simulink model "UDPVarFrameTest"  (R2013b)
settings: Solver=ode1  StartTime=0.0  StopTime=300  FixedStep=simPars.SampleTime  RelTol=1e-3
undefined symbols (not defined in the file or in its folder): simPars
libraries: instrumentlib x2, etargetslib x1
settings Model: Creator=Paul Freeman  LastModifiedBy=descobar
settings DataIOCC: LimitDataPoints=off  SignalLoggingSaveFormat=ModelDataLogs  SaveOutput=off  SignalLogging=off
settings OptimizationCC: ExpressionDepthLimit=2147483647
settings DebuggingCC: FcnCallInpInsideContextMsg=UseLocalSettings  StateNameClashWarn=warning
settings HardwareCC: ProdLargestAtomicInteger=Long  ProdLargestAtomicFloat=Double  ProdIntDivRoundTo=Zero  ProdEndianess=BigEndian  ProdHWDeviceType=Freescale->32-bit PowerPC
settings SFSimCC: SimParseCustomCode=off
settings GRTTargetCC: CombineOutputUpdateFcns=off  GRTInterface=on

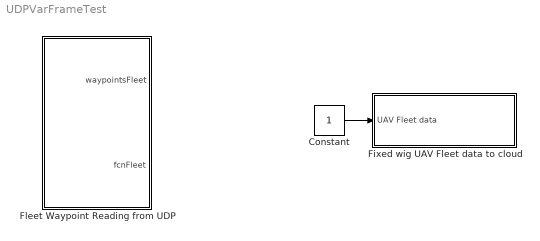
== system UDPVarFrameTest ==
  Constant : Constant
  Fixed wig UAV Fleet data to cloud : Subsystem
  Fleet Waypoint Reading from UDP : Subsystem
  wires:
  Constant/1 -> Fixed wig UAV Fleet data to cloud/1(UAV Fleet data)

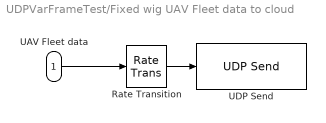
== system UDPVarFrameTest/Fixed wig UAV Fleet data to cloud ==
  UAV Fleet data : Inport
  Rate Transition : RateTransition  OutPortSampleTime=simPars.SampleTime*5
  UDP Send : instrumentlib/UDP Send  Host=localhost  Port=5556  LocalPort=5556  EnableBlockingMode=on  ByteOrder=BigEndian
  wires:
  Rate Transition/1 -> UDP Send/1
  UAV Fleet data/1 -> Rate Transition/1

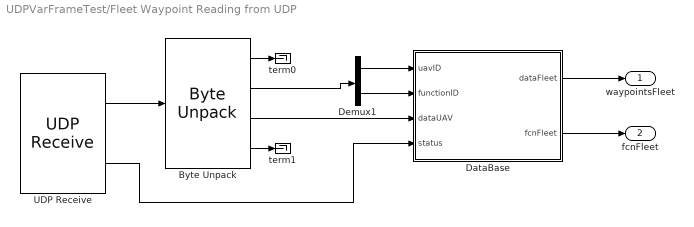
== system UDPVarFrameTest/Fleet Waypoint Reading from UDP ==
  Byte Unpack : etargetslib/Byte Unpack  dimensions={[3],[2],[30], [1]}  datatypes={'uint8', 'uint16', 'double','uint16'}  byteAlign=1
  "DataBase " : MATLAB Function  TreatAsAtomicUnit=on
  Demux1 : Demux  Outputs=2
  UDP Receive : instrumentlib/UDP Receive  Host=localhost  Port=9999  LocalPort=9999  DataSize="[249    1]"  EnableBlockingMode=off  Timeout=10  SampleTime=0.02  DataType=uint8  ByteOrder=BigEndian
  term0 : Terminator
  term1 : Terminator
  waypointsFleet : Outport
  fcnFleet : Outport  Port=2
  wires:
  "DataBase "/1(dataFleet) -> waypointsFleet/1
  Demux1/2 -> "DataBase "/2(functionID)
  UDP Receive/2 -> "DataBase "/4(status)
  Demux1/1 -> "DataBase "/1(uavID)
  Byte Unpack/3 -> "DataBase "/3(dataUAV)
  Byte Unpack/2 -> Demux1/1
  UDP Receive/1 -> Byte Unpack/1
  "DataBase "/2(fcnFleet) -> fcnFleet/1
  Byte Unpack/1 -> term0/1
  Byte Unpack/4 -> term1/1

== matlab function UDPVarFrameTest/Fleet Waypoint Reading from UDP/DataBase  ==
  data: uavID input; functionID input; dataUAV input; dataFleet output; fcnFleet output; status input
function [dataFleet,fcnFleet] = fcn(uavID, functionID , dataUAV, status)
%#codegen
nAC = 2; 
nWPs = 10; % maximum number of waypoints
%argument nAC; 

fcnFleet = zeros(nAC,1) ;

persistent waypointsFleet; 

if isempty(waypointsFleet)
    waypointsFleet = zeros(3,100, nAC);  
end

dataBytes = 155; 
udpHandle = udp('127.0.0.1',5554);
fopen(udpHandle) ;
fwrite(udpHandle,dataBytes);
fclose(udpHandle) ; 
delete(udpHandle) ;


switch functionID
    case 1 % setting waypoint list of a UAV into database
        if (uavID <= nAC )
            waypointsFleet(:,1:nWPs,uavID) = reshape(dataUAV, 3 ,nWPs  ); 
            if status ==1
                fcnFleet(uavID) =functionID ; % reset
                disp('status = 1') ;
            end
        end
        
        
    otherwise
        
        
    
end


dataFleet = waypointsFleet(1:3,:,:);
